simulink model "rlWalkingspotmini_ly"  (R2019a)
settings: Solver=ode113  StartTime=0.0  StopTime=Tf  FixedStep=0.025  RelTol=1e-1  EnableMultiTasking=on
values from neighbouring files (symbols this model uses):
  Tf = 10    [initializeRobotParameters.m]
  Ts = 0.025    [initializeRobotParameters.m]
undefined symbols (not defined in the file or in its folder): height_plane, init_angs_R, init_height, joint_stiffness, plane_x, plane_y, wx0, wy0, X, Y, Z
libraries: sm_lib x66, rlWalkingRobotUtils x20, nesl_utility x14, simulink x5, rllib x1, robotcorelib x1
(part 1 of 3)
settings Model: Creator=The MathWorks, Inc.  LastModifiedBy=liyan
settings SolverCC: ZeroCrossAlgorithm=Adaptive
settings DataIOCC: SaveOutput=off  SignalLogging=off  DSMLogging=off  SaveTime=off  ReturnWorkspaceOutputs=off  OutputTimes=0:0.01:10
settings OptimizationCC: LifeSpan=inf
settings DebuggingCC: AlgebraicLoopMsg=none  MaxConsecutiveZCsMsg=warning  IgnoredZcDiagnostic=none  AllowSymbolicDim=off  SFUnexpectedBacktrackingDiag=warning  SFNoUnconditionalDefaultTransitionDiag=warning  SFExecutionAtInitializationDiag=none  UnitsInconsistencyMsg=none  ArithmeticOperatorsInVariantConditions=warning
settings SFSimCC: SimUseLocalCustomCode=off
settings RTWCC: RTWUseLocalCustomCode=off
settings CodeAppCC: StateflowObjectComments=on
settings GRTTargetCC: TargetLangStandard=C89/C90 (ANSI)  GeneratePreprocessorConditionals=Disable all
settings ConfigComp: CovMetricSettings=dw  CovHtmlReporting=on  CovSaveCumulativeToWorkspaceVar=on  CovSaveSingleToWorkspaceVar=on  CovExternalEMLEnable=off  CovSFcnEnable=off
settings SimscapeCC: SimscapeNormalizeSystem=off  SimscapeLogOpenViewer=on  SimscapeLogLimitData=off  SimscapeLogDataHistory=10000
settings ConfigurationSet: Description=SimMechanics 2G
settings DiagnosticsConfigSet: SimMechanicsRigidlyBoundBlock=none
settings ExplorerConfigSet: InternalSimMechanicsExplorerSettings="<ExplorerConfiguration><canonicalview>default</canonicalview><AnimationSetting><BasePlaybackSpeed>1.0</BasePlaybackSpeed><PlaybackSpeedFactor>1.0</PlaybackSpeedFactor></AnimationSetting><TilePanel><TileInfo><Tiles Columns=\"1\" Count=\"1\" Rows=\"1\"><Column Weight=\"1\"/><Row Weight=\"1\"/><Tile Height=\"1\" Width=\"1\" X=\"0\" Y=\"0\"/></Tiles></TileInfo><SceneInfo><SceneViewer><BGColor><R>0.60000002384185791</R><G>0.60000002384185791</G><B>0.60000002384185791</B></BGColor><Camera><DoPerspective>off</DoPerspective><Position><X>7.18002534815406079</X><Y>-8.21011991112170847</Y><Z>8.33180938462712462</Z></Position><Center><X>1.10741005252516134</X><Y>-0.176829942633513204</Y><Z>0.646464709811595872</Z></Center><Up><X>-0.335329266167064488</X><Y>0.506481739462631531</Y><Z>0.79437430147428989</Z></Up><ViewLimDist>1</ViewLimDist><YLim>0.739205014828661411</YLim><XLim>1.12849377732657596</XLim></Camera></SceneViewer></SceneInfo></TilePanel><MechEditorPanel><Cameras/><GfxPanelCameraMap/><VideoCreator><PlaybackSpeedRatio>1.0</PlaybackSpeedRatio><FrameRate>30</FrameRate><VideoFormat>Motion JPEG AVI</VideoFormat><FrameSize>auto</FrameSize></VideoCreator></MechEditorPanel></ExplorerConfiguration>"

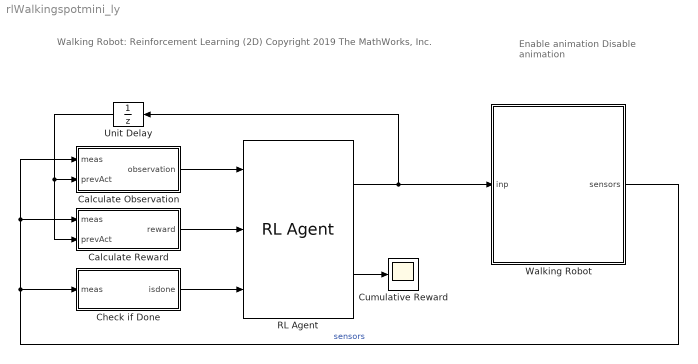
== system rlWalkingspotmini_ly ==
  note: Enable animation
      |
      | Disable animation
  note: Walking Robot: Reinforcement Learning (2D)
      |
      | Copyright 2019 The MathWorks, Inc.
  Calculate Observation : Subsystem
  Calculate Reward : Subsystem
  Check if Done : Subsystem
  Cumulative Reward : Scope
  RL Agent : rllib/RL Agent  Agent=agent  ProvideReward=on  ProvideIsDone=on  ProvideCumRwd=on  TreatAsDirectFeedthrough=on  CollectLoggedSignals=on  CollectModelStates=on
      settings: SourceProductName=Reinforcement Learning Toolbox
  Unit Delay : UnitDelay  SampleTime=-1  HasFrameUpgradeWarning=on
  Walking Robot : Subsystem
  wires:
  Walking Robot/1(sensors) -> Calculate Reward/1(meas), Calculate Observation/1(meas), Check if Done/1(meas)  "sensors"
  Calculate Reward/1(reward) -> RL Agent/2
  Calculate Observation/1(observation) -> RL Agent/1
  Check if Done/1(isdone) -> RL Agent/3
  RL Agent/2 -> Cumulative Reward/1
  Unit Delay/1 -> Calculate Reward/2(prevAct), Calculate Observation/2(prevAct)
  RL Agent/1 -> Walking Robot/1(inp), Unit Delay/1

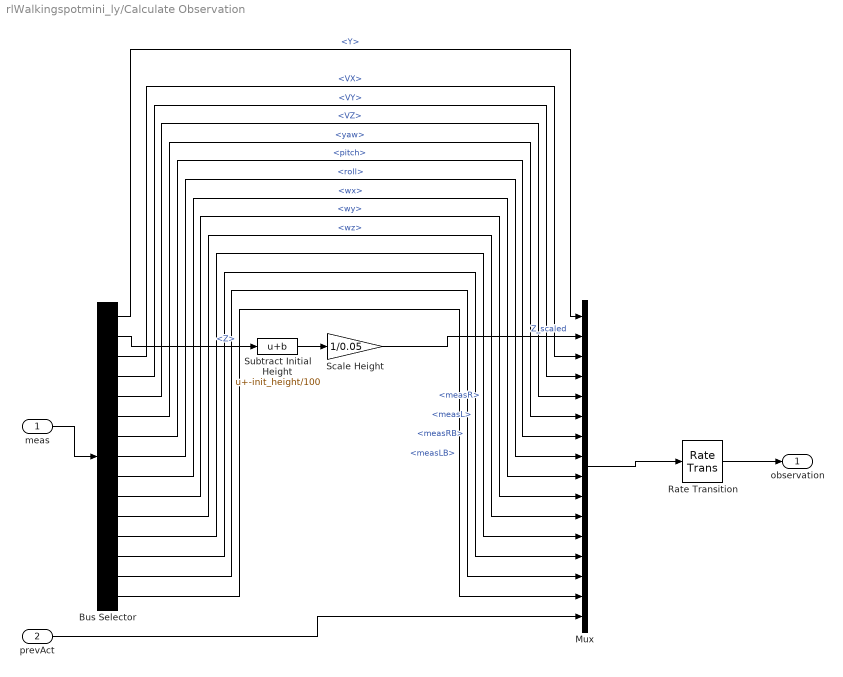
== system rlWalkingspotmini_ly/Calculate Observation ==
  meas : Inport
  prevAct : Inport  Port=2
  Bus Selector : BusSelector  OutputSignals=Y,Z,VX,VY,VZ,yaw,pitch,roll,wx,wy,wz,measR,measL,measRB,measLB
  Mux : Mux  Inputs=16
  Rate Transition : RateTransition
  Scale Height : Gain  Gain=1/0.05
  Subtract Initial Height : Bias  Bias=-init_height/100
  observation : Outport
  wires:
  meas/1 -> Bus Selector/1
  Mux/1 -> Rate Transition/1
  Rate Transition/1 -> observation/1
  Bus Selector/2 -> Subtract Initial Height/1  "<Z>"
  Subtract Initial Height/1 -> Scale Height/1
  Scale Height/1 -> Mux/2  "Z_scaled"
  Bus Selector/1 -> Mux/1  "<Y>"
  Bus Selector/4 -> Mux/4  "<VY>"
  Bus Selector/5 -> Mux/5  "<VZ>"
  Bus Selector/3 -> Mux/3  "<VX>"
  Bus Selector/6 -> Mux/6  "<yaw>"
  Bus Selector/7 -> Mux/7  "<pitch>"
  Bus Selector/8 -> Mux/8  "<roll>"
  Bus Selector/9 -> Mux/9  "<wx>"
  Bus Selector/10 -> Mux/10  "<wy>"
  Bus Selector/11 -> Mux/11  "<wz>"
  prevAct/1 -> Mux/16
  Bus Selector/12 -> Mux/12  "<measR>"
  Bus Selector/13 -> Mux/13  "<measL>"
  Bus Selector/14 -> Mux/14  "<measRB>"
  Bus Selector/15 -> Mux/15  "<measLB>"

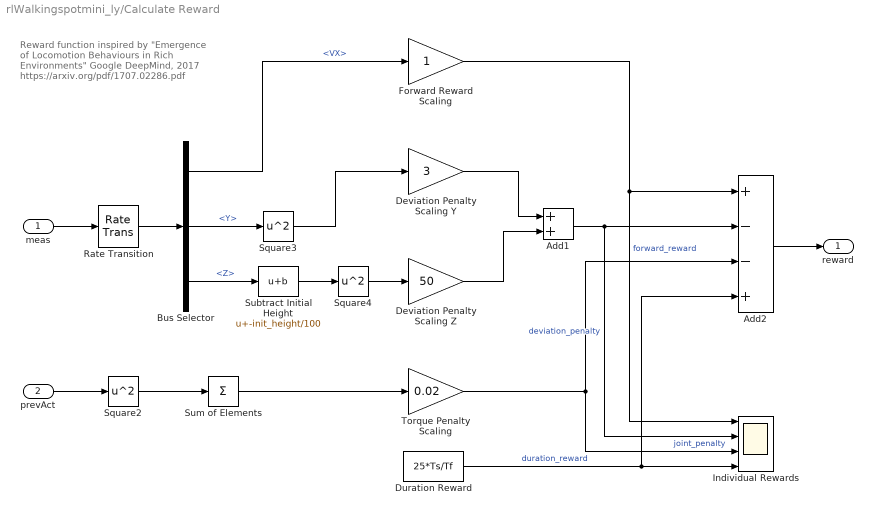
== system rlWalkingspotmini_ly/Calculate Reward ==
  note: Reward function inspired by
      | "Emergence of Locomotion Behaviours in Rich Environments"
      | Google DeepMind, 2017
      | https://arxiv.org/pdf/1707.02286.pdf
  meas : Inport
  prevAct : Inport  Port=2
  Add1 : Sum
  Add2 : Sum  Inputs=+--+
  Bus Selector : BusSelector  OutputSignals=VX,Y,Z
  Deviation Penalty Scaling Y : Gain  Gain=3
  Deviation Penalty Scaling Z : Gain  Gain=50
  Duration Reward : Constant  Value=25*Ts/Tf
  Forward Reward Scaling : Gain
  Individual Rewards : Scope  NumInputPorts=4
  Rate Transition : RateTransition  OutPortSampleTime=Ts
  Square2 : Math  Operator=square  SaturateOnIntegerOverflow=on
  Square3 : Math  Operator=square  SaturateOnIntegerOverflow=on
  Square4 : Math  Operator=square  SaturateOnIntegerOverflow=on
  Subtract Initial Height : Bias  Bias=-init_height/100
  Sum of Elements : Sum  Inputs=+
  Torque Penalty Scaling : Gain  Gain=0.02
  reward : Outport
  wires:
  meas/1 -> Rate Transition/1
  Rate Transition/1 -> Bus Selector/1
  Add2/1 -> reward/1
  Add1/1 -> Add2/2, Individual Rewards/2  "deviation_penalty"
  Forward Reward Scaling/1 -> Add2/1, Individual Rewards/1  "forward_reward"
  Sum of Elements/1 -> Torque Penalty Scaling/1
  Bus Selector/1 -> Forward Reward Scaling/1  "<VX>"
  Bus Selector/2 -> Square3/1  "<Y>"
  Square3/1 -> Deviation Penalty Scaling Y/1
  Duration Reward/1 -> Individual Rewards/4, Add2/4  "duration_reward"
  prevAct/1 -> Square2/1
  Square2/1 -> Sum of Elements/1
  Torque Penalty Scaling/1 -> Add2/3, Individual Rewards/3  "joint_penalty"
  Square4/1 -> Deviation Penalty Scaling Z/1
  Bus Selector/3 -> Subtract Initial Height/1  "<Z>"
  Subtract Initial Height/1 -> Square4/1
  Deviation Penalty Scaling Z/1 -> Add1/2
  Deviation Penalty Scaling Y/1 -> Add1/1

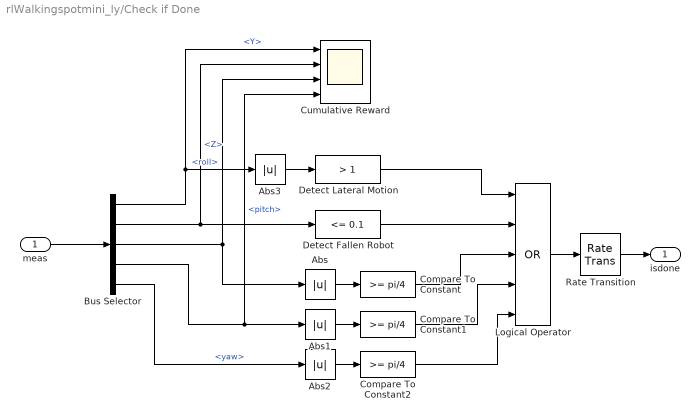
== system rlWalkingspotmini_ly/Check if Done ==
  meas : Inport
  Abs{,1..3} (4 alike) : Abs
  Bus Selector : BusSelector  OutputSignals=Y,Z,roll,pitch,yaw
  Compare To Constant : simulink/Logic and Bit Operations/Compare To Constant  relop=>=  const=pi/4  OutDataTypeStr=boolean
  Compare To Constant1 : simulink/Logic and Bit Operations/Compare To Constant  relop=>=  const=pi/4  OutDataTypeStr=boolean
  Compare To Constant2 : simulink/Logic and Bit Operations/Compare To Constant  relop=>=  const=pi/4  OutDataTypeStr=boolean
  Cumulative Reward : Scope  NumInputPorts=4
  Detect Fallen Robot : simulink/Logic and Bit Operations/Compare To Constant  relop=<=  const=0.1  OutDataTypeStr=boolean
  Detect Lateral Motion : simulink/Logic and Bit Operations/Compare To Constant  relop=>  const=1  OutDataTypeStr=boolean
  Logical Operator : Logic  Operator=OR  Inputs=5  AllPortsSameDT=off  OutDataTypeStr=boolean
  Rate Transition : RateTransition
  isdone : Outport
  wires:
  Logical Operator/1 -> Rate Transition/1
  Bus Selector/2 -> Cumulative Reward/2, Detect Fallen Robot/1  "<Z>"
  meas/1 -> Bus Selector/1
  Detect Fallen Robot/1 -> Logical Operator/2
  Bus Selector/3 -> Abs/1, Cumulative Reward/3  "<roll>"
  Bus Selector/4 -> Cumulative Reward/4, Abs1/1  "<pitch>"
  Compare To Constant/1 -> Logical Operator/3
  Abs/1 -> Compare To Constant/1
  Abs1/1 -> Compare To Constant1/1
  Compare To Constant1/1 -> Logical Operator/4
  Rate Transition/1 -> isdone/1
  Abs2/1 -> Compare To Constant2/1
  Bus Selector/5 -> Abs2/1  "<yaw>"
  Compare To Constant2/1 -> Logical Operator/5
  Abs3/1 -> Detect Lateral Motion/1
  Bus Selector/1 -> Cumulative Reward/1, Abs3/1  "<Y>"
  Detect Lateral Motion/1 -> Logical Operator/1

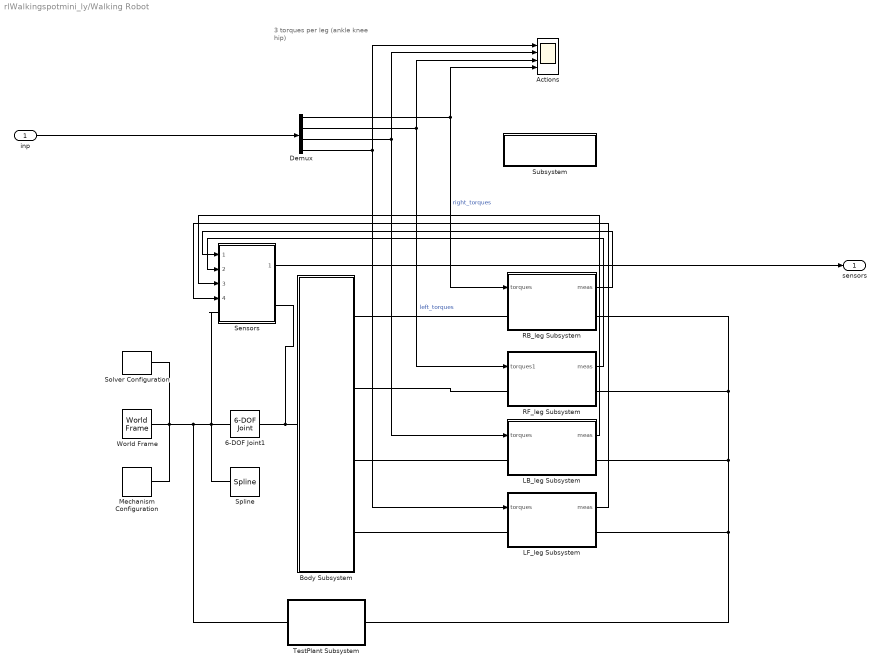
== system rlWalkingspotmini_ly/Walking Robot ==
  note: 3 torques per leg
      | (ankle knee hip)
  inp : Inport
  6-DOF Joint1 : sm_lib/Joints/6-DOF Joint  SenseConstraintForce=off  SenseConstraintForceX=off  SenseConstraintForceY=off  SenseConstraintForceZ=off  SenseConstraintTorque=off  SenseConstraintTorqueX=off  SenseConstraintTorqueY=off  SenseConstraintTorqueZ=off  SenseTotalForce=off  SenseTotalForceX=off  SenseTotalForceY=off  SenseTotalForceZ=off  SenseTotalTorque=off  SenseTotalTorqueX=off  SenseTotalTorqueY=off  SenseTotalTorqueZ=off  CompositeWrenchDir=FollowerOnBase  CompositeWrenchFrame=BaseFrame  PxEquilibriumPosition=0  PxEquilibriumPositionUnits=m  PxSpringStiffness=0  PxSpringStiffnessUnits=N/m  PxDampingCoefficient=world_damping  PxDampingCoefficientUnits=N/(m/s)  PxTorqueActuationMode=NoTorque  PxMotionActuationMode=ComputedMotion  PxSensePosition=off  PxSenseVelocity=off  PxSenseAcceleration=off  PxSenseTorqueForce=off  PxSenseLowerLimitTorqueForce=off  PxSenseUpperLimitTorqueForce=off  PxLowerLimitSpecify=off  PxLowerLimitBound=-1  PxLowerLimitBoundUnits=m  PxLowerLimitStiffness=1e6  PxLowerLimitStiffnessUnits=N/m  PxLowerLimitDamping=1e3  PxLowerLimitDampingUnits=N/(m/s)  PxLowerLimitTransitionRegionWidth=1e-4  PxLowerLimitTransitionRegionWidthUnits=m  PxUpperLimitSpecify=off  PxUpperLimitBound=1  PxUpperLimitBoundUnits=m  PxUpperLimitStiffness=1e6  PxUpperLimitStiffnessUnits=N/m  PxUpperLimitDamping=1e3  PxUpperLimitDampingUnits=N/(m/s)  PxUpperLimitTransitionRegionWidth=1e-4  PxUpperLimitTransitionRegionWidthUnits=m  PxPositionTargetSpecify=on  PxPositionTargetPriority=High  PxPositionTargetValue=0  PxPositionTargetValueUnits=m  PxVelocityTargetSpecify=on  PxVelocityTargetPriority=High  PxVelocityTargetValue=vx0  PxVelocityTargetValueUnits=m/s  PyEquilibriumPosition=0  PyEquilibriumPositionUnits=m  PySpringStiffness=0  PySpringStiffnessUnits=N/m  PyDampingCoefficient=world_damping  PyDampingCoefficientUnits=N/(m/s)  PyTorqueActuationMode=NoTorque  PyMotionActuationMode=ComputedMotion  PySensePosition=off  PySenseVelocity=off  PySenseAcceleration=off  PySenseTorqueForce=off  PySenseLowerLimitTorqueForce=off  PySenseUpperLimitTorqueForce=off  PyLowerLimitSpecify=off  PyLowerLimitBound=-1  PyLowerLimitBoundUnits=m  PyLowerLimitStiffness=1e6  PyLowerLimitStiffnessUnits=N/m  PyLowerLimitDamping=1e3  PyLowerLimitDampingUnits=N/(m/s)  PyLowerLimitTransitionRegionWidth=1e-4  PyLowerLimitTransitionRegionWidthUnits=m  PyUpperLimitSpecify=off  PyUpperLimitBound=1  PyUpperLimitBoundUnits=m  PyUpperLimitStiffness=1e6  PyUpperLimitStiffnessUnits=N/m  PyUpperLimitDamping=1e3  PyUpperLimitDampingUnits=N/(m/s)  PyUpperLimitTransitionRegionWidth=1e-4  PyUpperLimitTransitionRegionWidthUnits=m  PyPositionTargetSpecify=on  PyPositionTargetPriority=High  PyPositionTargetValue=0  PyPositionTargetValueUnits=m  PyVelocityTargetSpecify=on  PyVelocityTargetPriority=High  PyVelocityTargetValue=0  PyVelocityTargetValueUnits=m/s  PzEquilibriumPosition=0  PzEquilibriumPositionUnits=m  PzSpringStiffness=0  PzSpringStiffnessUnits=N/m  PzDampingCoefficient=world_damping  PzDampingCoefficientUnits=N/(m/s)  PzTorqueActuationMode=NoTorque  PzMotionActuationMode=ComputedMotion  PzSensePosition=off  PzSenseVelocity=off  PzSenseAcceleration=off  PzSenseTorqueForce=off  PzSenseLowerLimitTorqueForce=off  PzSenseUpperLimitTorqueForce=off  PzLowerLimitSpecify=off  PzLowerLimitBound=-1  PzLowerLimitBoundUnits=m  PzLowerLimitStiffness=1e6  PzLowerLimitStiffnessUnits=N/m  PzLowerLimitDamping=1e3  PzLowerLimitDampingUnits=N/(m/s)  PzLowerLimitTransitionRegionWidth=1e-4  PzLowerLimitTransitionRegionWidthUnits=m  PzUpperLimitSpecify=off  PzUpperLimitBound=1  PzUpperLimitBoundUnits=m  PzUpperLimitStiffness=1e6  PzUpperLimitStiffnessUnits=N/m  PzUpperLimitDamping=1e3  PzUpperLimitDampingUnits=N/(m/s)  PzUpperLimitTransitionRegionWidth=1e-4  PzUpperLimitTransitionRegionWidthUnits=m  PzPositionTargetSpecify=on  PzPositionTargetPriority=High  PzPositionTargetValue=init_height  PzPositionTargetValueUnits=cm  PzVelocityTargetSpecify=off  PzVelocityTargetPriority=High  PzVelocityTargetValue=0  PzVelocityTargetValueUnits=m/s  SphDefPosRotationMethod=None  SphDefPosRotationAngleUnits=deg  SphDefPosRotationStandardAxis=+Z  SphDefPosRotationAngle=0.0  SphDefPosRotationArbitraryAxis=[0 0 1]  SphDefPosFollAlignAxisA=+X  SphDefPosBaseAlignAxisA=+Y  SphDefPosFollAlignAxisB=+Y  SphDefPosBaseAlignAxisB=+Z  SphDefPosRotationSequenceAxes=FollowerAxes  SphDefPosRotationSequence=XYX  SphDefPosRotationSequenceAngles=[0 0 0]  SphDefPosRotationSequenceAnglesUnits=deg  SphDefPosRotationMatrix=[1 0 0; 0 1 0; 0 0 1]  SphEqPosRotationMethod=None  SphEqPosRotationAngleUnits=deg  SphEqPosRotationStandardAxis=+Z  SphEqPosRotationAngle=0.0  SphEqPosRotationArbitraryAxis=[0 0 1]  SphEqPosFollAlignAxisA=+X  SphEqPosBaseAlignAxisA=+Y  SphEqPosFollAlignAxisB=+Y  SphEqPosBaseAlignAxisB=+Z  SphEqPosRotationSequenceAxes=FollowerAxes  SphEqPosRotationSequence=XYX  SphEqPosRotationSequenceAngles=[0 0 0]  SphEqPosRotationSequenceAnglesUnits=deg  SphEqPosRotationMatrix=[1 0 0; 0 1 0; 0 0 1]  SphSpringStiffness=0  SphSpringStiffnessUnits=N*m/deg  SphDampingCoefficient=world_rot_damping  SphDampingCoefficientUnits=N*m/(rad/s)  SphActuateTorqueX=off  SphActuateTorqueY=off  SphActuateTorqueZ=off  SphActuateTorque=off  SphTorqueActuationMode=NoTorque  SphMotionActuationMode=ComputedMotion  SphActuationFrame=BaseFrame  SphSensePosition=off  SphSenseVelocityX=off  SphSenseVelocityY=off  SphSenseVelocityZ=off  SphSenseVelocity=off  SphSenseAccelerationX=off  SphSenseAccelerationY=off  SphSenseAccelerationZ=off  SphSenseAcceleration=off  SphSenseTorqueX=off  SphSenseTorqueY=off  SphSenseTorqueZ=off  SphSenseTorqueForce=off  SphSenseLowerLimitTorqueMag=off  SphSenseUpperLimitTorqueMag=off  SphSensingFrame=BaseFrame  SphLowerLimitSpecify=off  SphLowerLimitBound=15  SphLowerLimitBoundUnits=deg  SphLowerLimitStiffness=1e4  SphLowerLimitStiffnessUnits=N*m/deg  SphLowerLimitDamping=10  SphLowerLimitDampingUnits=N*m/(deg/s)  SphLowerLimitTransitionRegionWidth=0.1  SphLowerLimitTransitionRegionWidthUnits=deg  SphUpperLimitSpecify=off  SphUpperLimitBound=45  SphUpperLimitBoundUnits=deg  SphUpperLimitStiffness=1e4  SphUpperLimitStiffnessUnits=N*m/deg  SphUpperLimitDamping=10  SphUpperLimitDampingUnits=N*m/(deg/s)  SphUpperLimitTransitionRegionWidth=0.1  SphUpperLimitTransitionRegionWidthUnits=deg  SphPositionTargetRotationMethod=RotationSequence  SphPositionTargetRotationAngleUnits=deg  SphPositionTargetRotationStandardAxis=+Z  SphPositionTargetRotationAngle=0.0  SphPositionTargetRotationArbitraryAxis=[0 0 1]  SphPositionTargetFollAlignAxisA=+X  SphPositionTargetBaseAlignAxisA=+Y  SphPositionTargetFollAlignAxisB=+Y  SphPositionTargetBaseAlignAxisB=+Z  SphPositionTargetRotationSequenceAxes=FollowerAxes  SphPositionTargetRotationSequence=XYX  SphPositionTargetRotationSequenceAngles=[wx0 wy0 0]  SphPositionTargetRotationSequenceAnglesUnits=rad  SphPositionTargetRotationMatrix=eye(3)  SphPositionTargetSpecify=on  SphPositionTargetPriority=High  SphVelocityTargetValue=[0 0 0]  SphVelocityTargetValueUnits=deg/s  SphVelocityTargetSpecify=off  SphVelocityTargetPriority=High  SphVelocityTargetInFollowerFrame=on
  Actions : Scope  NumInputPorts=4
  Body Subsystem : Subsystem
  Demux : Demux
  LB_leg Subsystem : Subsystem
  LF_leg Subsystem : Subsystem
  Mechanism Configuration : sm_lib/Utilities/Mechanism Configuration  UniformGravity=Constant  GravityVector=[0 0 -9.80665]  GravityUnits=m/s^2  LinearizationDelta=0.001
  RB_leg Subsystem : Subsystem
  RF_leg Subsystem : Subsystem
  Sensors : Subsystem
  Solver Configuration : nesl_utility/Solver Configuration  PhysicalDomain=network_engine_domain  SubClassName=solver  LeftPortType=input  RightPortType=generic  Tones=[]  Harmonics=[]  SimulateNoise=off  Profile=off  UseLocalSampling=off  EnableSwitchedLinearOptims=on  FrequencyDomain=off  UseCCode=off  RelTol=0.001  AbsTol=1e-06  MinStep=1e-09  ToWorkspace=off  RevertToSquareIcSolve=off  NumHomotopyIterations=100  PhasorMode=off  PhasorModeNumHarmonics=1  DoDC=off  ResidualTolerance=1e-09  UseLocalSolver=off  LocalSolverChoice=NE_BACKWARD_EULER_ADVANCER  LocalSolverSampleTime=0.001  DoFixedCost=off  MaxNonlinIter=3  MaxModeIter=2  LinearAlgebra=Sparse  EquationFormulation=NE_TIME_EF  DelaysMemoryBudget=1024  AutomaticFiltering=on  FilteringTimeConstant=0.001  PartitionStorageMethod=AS_NEEDED  PartitionMemoryBudget=1024  PartitionMethod=FAST
  Spline : sm_lib/Curves and Surfaces/Spline  DataPoints=[0 0 0.025; 5 0 0.025]  DataPointsUnits=m  EndConditionType=Natural  GraphicType=FromGeometry  MarkerShape=Sphere  MarkerSize=10  GraphicVisPropType=SimpleVisualProperties  GraphicDiffuseColor=[0 0 0]  GraphicSpecularColor=[0.5 0.5 0.5 1.0]  GraphicAmbientColor=[0.15 0.15 0.15 1.0]  GraphicEmissiveColor=[0.0 0.0 0.0 1.0]  GraphicShininess=75  GraphicOpacity=1.0
      settings: SourceProductName=Simscape Multibody
  Subsystem : Subsystem
      settings: OpenFcn=open_system('sm_lib')
      mask Display: disp(sprintf('Open Simscape Multibody\nLibrary'));
  TestPlant Subsystem : Subsystem
  World Frame : sm_lib/Frames and Transforms/World Frame
  sensors : Outport
  wires:
  Demux/3 -> LB_leg Subsystem/1(torques), Actions/2
  Demux/1 -> RB_leg Subsystem/1(torques), Actions/4  "right_torques"
  RF_leg Subsystem/1(meas) -> Sensors/2(measRB)
  Demux/4 -> LF_leg Subsystem/1(torques), Actions/1
  LB_leg Subsystem/1(meas) -> Sensors/3(measLF)
  LF_leg Subsystem/1(meas) -> Sensors/4(measLB)
  Demux/2 -> RF_leg Subsystem/1(torques1), Actions/3  "left_torques"
  Sensors/1(sensors) -> sensors/1
  inp/1 -> Demux/1
  RB_leg Subsystem/1(meas) -> Sensors/1(measRF)
  connections:
  TestPlant Subsystem/RConn1 -- RB_leg Subsystem/RConn1 -- RF_leg Subsystem/RConn1 -- LB_leg Subsystem/RConn1 -- LF_leg Subsystem/RConn1
  TestPlant Subsystem/LConn1 -- World Frame/RConn1 -- Mechanism Configuration/RConn1 -- Solver Configuration/RConn1 -- 6-DOF Joint1/LConn1 -- Spline/LConn1 -- Sensors/LConn1
  Body Subsystem/LConn1 -- 6-DOF Joint1/RConn1 -- Sensors/RConn1
  RB_leg Subsystem/LConn1 -- Body Subsystem/RConn1
  Body Subsystem/RConn4 -- LF_leg Subsystem/LConn1
  RF_leg Subsystem/LConn1 -- Body Subsystem/RConn2
  Body Subsystem/RConn3 -- LB_leg Subsystem/LConn1

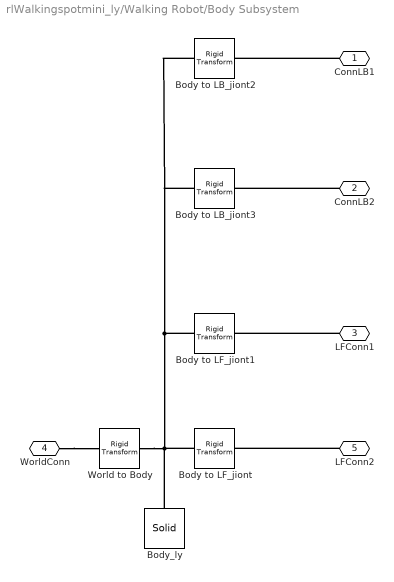
== system rlWalkingspotmini_ly/Walking Robot/Body Subsystem ==
  Body to LB_jiont2 : sm_lib/Frames and Transforms/Rigid Transform  TranslationMethod=Cartesian  TranslationStandardOffset=100  TranslationLengthUnit=mm  TranslationStandardAxis=+Z  TranslationCartesianOffset=[-40 -115 6.5]  TranslationROffset=0  TranslationROffsetUnits=m  TranslationZOffset=0  TranslationZOffsetUnits=m  TranslationThetaOffset=0  TranslationThetaOffsetUnits=deg  RotationMethod=StandardAxis  RotationAngleUnits=deg  RotationStandardAxis=+X  RotationAngle=90  RotationArbitraryAxis=[0 0 1]  FollAlignAxisA=+Z  BaseAlignAxisA=+X  FollAlignAxisB=+Y  BaseAlignAxisB=+Z  RotationSequenceAxes=FollowerAxes  RotationSequence=XYX  RotationSequenceAngles=[0 0 0]  RotationSequenceAnglesUnits=deg  RotationMatrix=[1 0 0; 0 1 0; 0 0 1]
  Body to LB_jiont3 : sm_lib/Frames and Transforms/Rigid Transform  TranslationMethod=Cartesian  TranslationStandardOffset=100  TranslationLengthUnit=mm  TranslationStandardAxis=+Z  TranslationCartesianOffset=[-40 70 6.5]  TranslationROffset=0  TranslationROffsetUnits=m  TranslationZOffset=0  TranslationZOffsetUnits=m  TranslationThetaOffset=0  TranslationThetaOffsetUnits=deg  RotationMethod=StandardAxis  RotationAngleUnits=deg  RotationStandardAxis=+X  RotationAngle=90  RotationArbitraryAxis=[0 0 1]  FollAlignAxisA=+Z  BaseAlignAxisA=+X  FollAlignAxisB=+Y  BaseAlignAxisB=+Z  RotationSequenceAxes=FollowerAxes  RotationSequence=XYX  RotationSequenceAngles=[0 0 0]  RotationSequenceAnglesUnits=deg  RotationMatrix=[1 0 0; 0 1 0; 0 0 1]
  Body to LF_jiont : sm_lib/Frames and Transforms/Rigid Transform  TranslationMethod=Cartesian  TranslationStandardOffset=100  TranslationLengthUnit=mm  TranslationStandardAxis=+Z  TranslationCartesianOffset=[40 70 6.5]  TranslationROffset=0  TranslationROffsetUnits=m  TranslationZOffset=0  TranslationZOffsetUnits=m  TranslationThetaOffset=0  TranslationThetaOffsetUnits=deg  RotationMethod=StandardAxis  RotationAngleUnits=deg  RotationStandardAxis=+X  RotationAngle=90  RotationArbitraryAxis=[0 0 1]  FollAlignAxisA=+Z  BaseAlignAxisA=+X  FollAlignAxisB=+Y  BaseAlignAxisB=+Z  RotationSequenceAxes=FollowerAxes  RotationSequence=XYX  RotationSequenceAngles=[0 0 0]  RotationSequenceAnglesUnits=deg  RotationMatrix=[1 0 0; 0 1 0; 0 0 1]
  Body to LF_jiont1 : sm_lib/Frames and Transforms/Rigid Transform  TranslationMethod=Cartesian  TranslationStandardOffset=100  TranslationLengthUnit=mm  TranslationStandardAxis=+Z  TranslationCartesianOffset=[40 -115 6.5]  TranslationROffset=0  TranslationROffsetUnits=m  TranslationZOffset=0  TranslationZOffsetUnits=m  TranslationThetaOffset=0  TranslationThetaOffsetUnits=deg  RotationMethod=StandardAxis  RotationAngleUnits=deg  RotationStandardAxis=+X  RotationAngle=90  RotationArbitraryAxis=[0 0 1]  FollAlignAxisA=+Z  BaseAlignAxisA=+X  FollAlignAxisB=+Y  BaseAlignAxisB=+Z  RotationSequenceAxes=FollowerAxes  RotationSequence=XYX  RotationSequenceAngles=[0 0 0]  RotationSequenceAnglesUnits=deg  RotationMatrix=[1 0 0; 0 1 0; 0 0 1]
  Body_ly : sm_lib/Body Elements/Solid  InertiaType=Custom  Mass=100  MassUnits=g  CenterOfMass=[0 0 0]  CenterOfMassUnits=mm  MomentsOfInertia=[1 1 1]  MomentsOfInertiaUnits=kg*m^2  ProductsOfInertia=[0 0 0]  ProductsOfInertiaUnits=kg*m^2  BasedOnType=Density  Density=1000  DensityUnits=kg/m^3  DoExposeReferenceFrame=on  SerializedFrames=<Frames/>  GraphicType=FromGeometry  MarkerShape=Sphere  MarkerSize=10  GraphicVisPropType=SimpleVisualProperties  GraphicDiffuseColor=[0.5 0.5 0.5]  GraphicSpecularColor=[0.5 0.5 0.5 1.0]  GraphicAmbientColor=[0.15 0.15 0.15 1.0]  GraphicEmissiveColor=[0.0 0.0 0.0 1.0]  GraphicShininess=75  GraphicOpacity=1.0  GeometryShape=FromFile  RectangleSize=[1 1]  RectangleSizeUnits=m  BrickDimensions=[1 1 1]  BrickDimensionUnits=m  CylinderRadius=1  CylinderRadiusUnits=m  CylinderLength=1  CylinderLengthUnits=m  SphereRadius=1  SphereRadiusUnits=m  EllipsoidRadii=[1 1 1]  EllipsoidRadiiUnits=m  ExtrusionCrossSection=[1 1; -1 1; -1 -1; 1 -1]  ExtrusionCrossSectionUnits=m  ExtrusionLength=1  ExtrusionLengthUnits=m  PolygonNumSides=3  PolygonOuterRadius=1  PolygonOuterRadiusUnits=m  ExtGeomFileType=STL  ExtGeomFileName=D:\MATLAB\robota\sportmicro\sportmicro\body_ly.STL  ExtGeomFileUnits=mm  RevolutionCrossSection=[1 1; 1 -1; 2 -1; 2 1]  RevolutionCrossSectionUnits=m  RevolutionExtent=Full  RevolutionAngle=180  RevolutionAngleUnits=deg
  World to Body : sm_lib/Frames and Transforms/Rigid Transform  TranslationMethod=Cartesian  TranslationStandardOffset=100  TranslationLengthUnit=mm  TranslationStandardAxis=+Z  TranslationCartesianOffset=[0 0 50]  TranslationROffset=0  TranslationROffsetUnits=m  TranslationZOffset=0  TranslationZOffsetUnits=m  TranslationThetaOffset=0  TranslationThetaOffsetUnits=deg  RotationMethod=AlignedAxes  RotationAngleUnits=deg  RotationStandardAxis=+X  RotationAngle=180  RotationArbitraryAxis=[0 0 1]  FollAlignAxisA=+Z  BaseAlignAxisA=-Z  FollAlignAxisB=-X  BaseAlignAxisB=-Y  RotationSequenceAxes=BaseAxes  RotationSequence=XYX  RotationSequenceAngles=[180 0 0]  RotationSequenceAnglesUnits=deg  RotationMatrix=[1 0 0; 0 1 0; 0 0 1]
  ConnLB1 : PMIOPort  Side=Right
  ConnLB2 : PMIOPort  Port=2  Side=Right
  LFConn1 : PMIOPort  Port=3  Side=Right
  WorldConn : PMIOPort  Port=4  Side=Left
  LFConn2 : PMIOPort  Port=5  Side=Right
  connections:
  LFConn2/RConn1 -- Body to LF_jiont/RConn1
  Body_ly/RConn1 -- Body to LB_jiont3/LConn1 -- Body to LB_jiont2/LConn1 -- Body to LF_jiont1/LConn1 -- World to Body/RConn1 -- Body to LF_jiont/LConn1
  LFConn1/RConn1 -- Body to LF_jiont1/RConn1
  WorldConn/RConn1 -- World to Body/LConn1
  ConnLB2/RConn1 -- Body to LB_jiont3/RConn1
  ConnLB1/RConn1 -- Body to LB_jiont2/RConn1

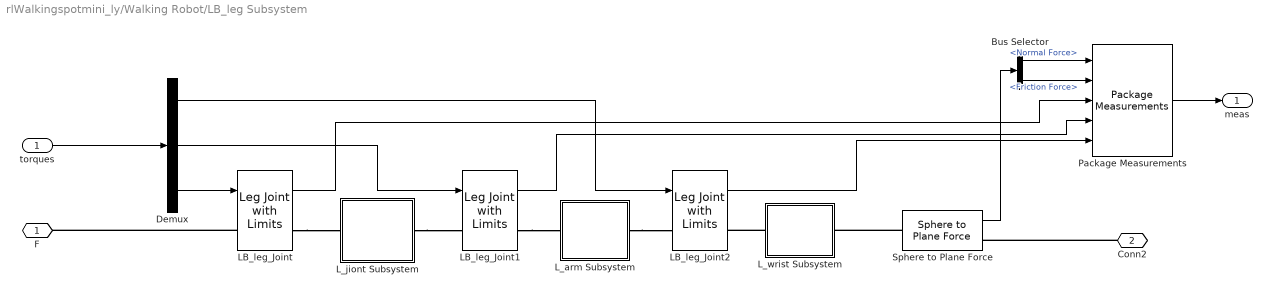
== system rlWalkingspotmini_ly/Walking Robot/LB_leg Subsystem ==
  torques : Inport
  Bus Selector : BusSelector  OutputSignals=Normal Force,Friction Force
  Demux : Demux  Outputs=3
  LB_leg_Joint : rlWalkingRobotUtils/Leg Joint with Limits  VariantControl=actuatorType == 2  k=joint_stiffness  d=joint_damping  initAngle=0%init_angs_R(2)  eqAngle=0  upperLimit=pi  lowerLimit=0  jointLimitStiffness=joint_limit_stiffness  jointLimitDamping=joint_limit_damping
  LB_leg_Joint1 : rlWalkingRobotUtils/Leg Joint with Limits  VariantControl=actuatorType == 2  k=joint_stiffness  d=joint_damping  initAngle=0%init_angs_R(2)  eqAngle=0  upperLimit=pi  lowerLimit=0  jointLimitStiffness=joint_limit_stiffness  jointLimitDamping=joint_limit_damping
  LB_leg_Joint2 : rlWalkingRobotUtils/Leg Joint with Limits  VariantControl=actuatorType == 2  k=joint_stiffness  d=joint_damping  initAngle=0%init_angs_R(2)  eqAngle=0  upperLimit=pi  lowerLimit=0  jointLimitStiffness=joint_limit_stiffness  jointLimitDamping=joint_limit_damping
  L_arm Subsystem : Subsystem
  L_jiont Subsystem : Subsystem
  L_wrist Subsystem : Subsystem
  Package Measurements : rlWalkingRobotUtils/Package  Measurements  SystemSampleTime=-1
  Sphere to Plane Force : rlWalkingRobotUtils/Sphere to Plane Force  sphere_rad=contact_point_radius  plane_lenx=plane_x  plane_leny=plane_y  plane_depth=height_plane/2  force_law=Linear  k_contact=contact_stiffness  b_contact=contact_damping  pen_full_damp_F=1e-4  pen_exponent=1  custom_param_1=1  custom_param_2=1  friction_law=Stick-Slip Continuous  mu_kinetic=mu_k  mu_static=mu_s  v_thr=mu_vth  vis_on=on  vis_opc_en=0  vis_len_plaBz=0.005  vis_clr=[0.9 0.2 0.2]  vis_opc=0.7
  F : PMIOPort  Side=Left
  Conn2 : PMIOPort  Port=2  Side=Right
  meas : Outport
  wires:
  torques/1 -> Demux/1
  Demux/3 -> LB_leg_Joint/1
  Demux/2 -> LB_leg_Joint1/1
  Demux/1 -> LB_leg_Joint2/1
  Bus Selector/1 -> Package Measurements/1  "<Normal Force>"
  Sphere to Plane Force/1 -> Bus Selector/1
  Package Measurements/1 -> meas/1
  Bus Selector/2 -> Package Measurements/2  "<Friction Force>"
  LB_leg_Joint/1 -> Package Measurements/3
  LB_leg_Joint1/1 -> Package Measurements/4
  LB_leg_Joint2/1 -> Package Measurements/5
  connections:
  LB_leg_Joint1/RConn1 -- L_arm Subsystem/LConn1
  L_arm Subsystem/RConn1 -- LB_leg_Joint2/LConn1
  L_jiont Subsystem/RConn1 -- LB_leg_Joint1/LConn1
  L_wrist Subsystem/LConn1 -- LB_leg_Joint2/RConn1
  LB_leg_Joint/LConn1 -- F/RConn1
  LB_leg_Joint/RConn1 -- L_jiont Subsystem/LConn1
  Sphere to Plane Force/LConn1 -- L_wrist Subsystem/RConn1
  Conn2/RConn1 -- Sphere to Plane Force/RConn1

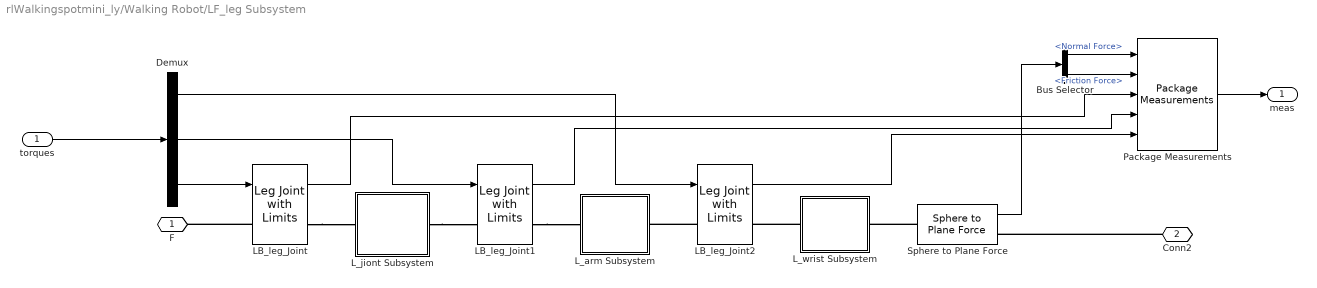
== system rlWalkingspotmini_ly/Walking Robot/LF_leg Subsystem ==
  torques : Inport
  Bus Selector : BusSelector  OutputSignals=Normal Force,Friction Force
  Demux : Demux  Outputs=3
  LB_leg_Joint : rlWalkingRobotUtils/Leg Joint with Limits  VariantControl=actuatorType == 2  k=joint_stiffness  d=joint_damping  initAngle=0%init_angs_R(2)  eqAngle=0  upperLimit=pi  lowerLimit=0  jointLimitStiffness=joint_limit_stiffness  jointLimitDamping=joint_limit_damping
  LB_leg_Joint1 : rlWalkingRobotUtils/Leg Joint with Limits  VariantControl=actuatorType == 2  k=joint_stiffness  d=joint_damping  initAngle=0%init_angs_R(2)  eqAngle=0  upperLimit=pi  lowerLimit=0  jointLimitStiffness=joint_limit_stiffness  jointLimitDamping=joint_limit_damping
  LB_leg_Joint2 : rlWalkingRobotUtils/Leg Joint with Limits  VariantControl=actuatorType == 2  k=joint_stiffness  d=joint_damping  initAngle=0%init_angs_R(2)  eqAngle=0  upperLimit=pi  lowerLimit=0  jointLimitStiffness=joint_limit_stiffness  jointLimitDamping=joint_limit_damping
  L_arm Subsystem : Subsystem
  L_jiont Subsystem : Subsystem
  L_wrist Subsystem : Subsystem
  Package Measurements : rlWalkingRobotUtils/Package  Measurements  SystemSampleTime=-1
  Sphere to Plane Force : rlWalkingRobotUtils/Sphere to Plane Force  sphere_rad=contact_point_radius  plane_lenx=plane_x  plane_leny=plane_y  plane_depth=height_plane/2  force_law=Linear  k_contact=contact_stiffness  b_contact=contact_damping  pen_full_damp_F=1e-4  pen_exponent=1  custom_param_1=1  custom_param_2=1  friction_law=Stick-Slip Continuous  mu_kinetic=mu_k  mu_static=mu_s  v_thr=mu_vth  vis_on=on  vis_opc_en=0  vis_len_plaBz=0.005  vis_clr=[0.9 0.2 0.2]  vis_opc=0.7
  F : PMIOPort  Side=Left
  Conn2 : PMIOPort  Port=2  Side=Right
  meas : Outport
  wires:
  torques/1 -> Demux/1
  Demux/3 -> LB_leg_Joint/1
  Demux/2 -> LB_leg_Joint1/1
  Demux/1 -> LB_leg_Joint2/1
  Bus Selector/1 -> Package Measurements/1  "<Normal Force>"
  Sphere to Plane Force/1 -> Bus Selector/1
  Package Measurements/1 -> meas/1
  Bus Selector/2 -> Package Measurements/2  "<Friction Force>"
  LB_leg_Joint/1 -> Package Measurements/3
  LB_leg_Joint1/1 -> Package Measurements/4
  LB_leg_Joint2/1 -> Package Measurements/5
  connections:
  LB_leg_Joint/LConn1 -- F/RConn1
  L_wrist Subsystem/LConn1 -- LB_leg_Joint2/RConn1
  L_jiont Subsystem/RConn1 -- LB_leg_Joint1/LConn1
  LB_leg_Joint2/LConn1 -- L_arm Subsystem/RConn1
  LB_leg_Joint1/RConn1 -- L_arm Subsystem/LConn1
  LB_leg_Joint/RConn1 -- L_jiont Subsystem/LConn1
  Sphere to Plane Force/LConn1 -- L_wrist Subsystem/RConn1
  Conn2/RConn1 -- Sphere to Plane Force/RConn1

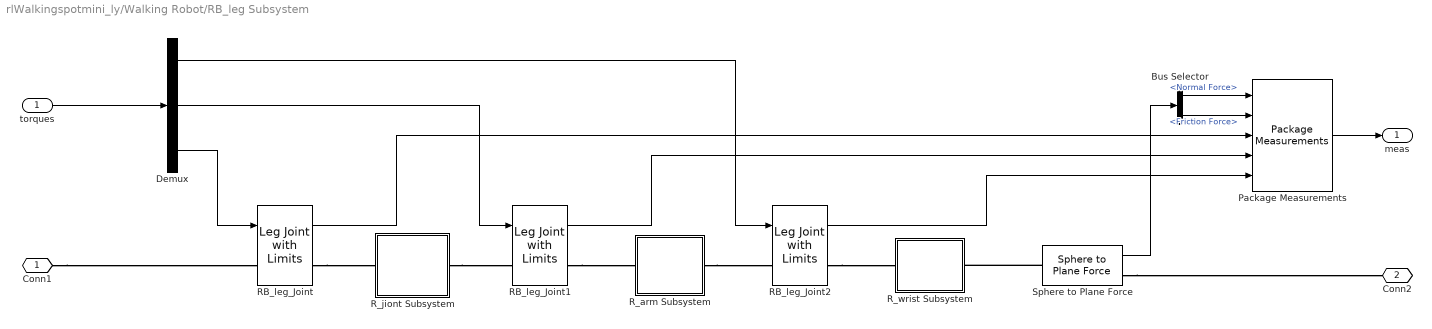
== system rlWalkingspotmini_ly/Walking Robot/RB_leg Subsystem ==
  torques : Inport
  Bus Selector : BusSelector  OutputSignals=Normal Force,Friction Force
  Demux : Demux  Outputs=3
  Package Measurements : rlWalkingRobotUtils/Package  Measurements  SystemSampleTime=-1
  RB_leg_Joint : rlWalkingRobotUtils/Leg Joint with Limits  VariantControl=actuatorType == 2  k=joint_stiffness  d=joint_damping  initAngle=0%init_angs_R(2)  eqAngle=0  upperLimit=pi  lowerLimit=0  jointLimitStiffness=joint_limit_stiffness  jointLimitDamping=joint_limit_damping
  RB_leg_Joint1 : rlWalkingRobotUtils/Leg Joint with Limits  VariantControl=actuatorType == 2  k=joint_stiffness  d=joint_damping  initAngle=0%init_angs_R(2)  eqAngle=0  upperLimit=pi  lowerLimit=0  jointLimitStiffness=joint_limit_stiffness  jointLimitDamping=joint_limit_damping
  RB_leg_Joint2 : rlWalkingRobotUtils/Leg Joint with Limits  VariantControl=actuatorType == 2  k=joint_stiffness  d=joint_damping  initAngle=0%init_angs_R(2)  eqAngle=0  upperLimit=pi  lowerLimit=0  jointLimitStiffness=joint_limit_stiffness  jointLimitDamping=joint_limit_damping
  R_arm Subsystem : Subsystem
  R_jiont Subsystem : Subsystem
  R_wrist Subsystem : Subsystem
  Sphere to Plane Force : rlWalkingRobotUtils/Sphere to Plane Force  sphere_rad=contact_point_radius  plane_lenx=plane_x  plane_leny=plane_y  plane_depth=height_plane/2  force_law=Linear  k_contact=contact_stiffness  b_contact=contact_damping  pen_full_damp_F=1e-4  pen_exponent=1  custom_param_1=1  custom_param_2=1  friction_law=Stick-Slip Continuous  mu_kinetic=mu_k  mu_static=mu_s  v_thr=mu_vth  vis_on=on  vis_opc_en=0  vis_len_plaBz=0.005  vis_clr=[0.9 0.2 0.2]  vis_opc=0.7
  Conn1 : PMIOPort  Side=Left
  Conn2 : PMIOPort  Port=2  Side=Right
  meas : Outport
  wires:
  Demux/3 -> RB_leg_Joint/1
  Demux/2 -> RB_leg_Joint1/1
  Demux/1 -> RB_leg_Joint2/1
  torques/1 -> Demux/1
  Package Measurements/1 -> meas/1
  Sphere to Plane Force/1 -> Bus Selector/1
  Bus Selector/1 -> Package Measurements/1  "<Normal Force>"
  Bus Selector/2 -> Package Measurements/2  "<Friction Force>"
  RB_leg_Joint/1 -> Package Measurements/3
  RB_leg_Joint1/1 -> Package Measurements/4
  RB_leg_Joint2/1 -> Package Measurements/5
  connections:
  RB_leg_Joint1/RConn1 -- R_arm Subsystem/LConn1
  R_arm Subsystem/RConn1 -- RB_leg_Joint2/LConn1
  RB_leg_Joint2/RConn1 -- R_wrist Subsystem/LConn1
  Conn1/RConn1 -- RB_leg_Joint/LConn1
  RB_leg_Joint/RConn1 -- R_jiont Subsystem/LConn1
  R_jiont Subsystem/RConn1 -- RB_leg_Joint1/LConn1
  Sphere to Plane Force/LConn1 -- R_wrist Subsystem/RConn1
  Sphere to Plane Force/RConn1 -- Conn2/RConn1

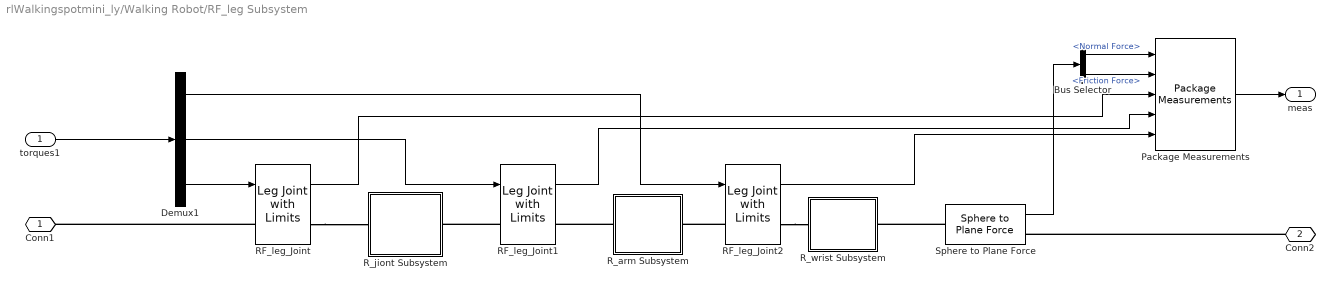
== system rlWalkingspotmini_ly/Walking Robot/RF_leg Subsystem ==
  torques1 : Inport
  Bus Selector : BusSelector  OutputSignals=Normal Force,Friction Force
  Demux1 : Demux  Outputs=3
  Package Measurements : rlWalkingRobotUtils/Package  Measurements  SystemSampleTime=-1
  RF_leg_Joint : rlWalkingRobotUtils/Leg Joint with Limits  VariantControl=actuatorType == 2  k=joint_stiffness  d=joint_damping  initAngle=0%init_angs_R(2)  eqAngle=0  upperLimit=pi  lowerLimit=0  jointLimitStiffness=joint_limit_stiffness  jointLimitDamping=joint_limit_damping
  RF_leg_Joint1 : rlWalkingRobotUtils/Leg Joint with Limits  VariantControl=actuatorType == 2  k=joint_stiffness  d=joint_damping  initAngle=0%init_angs_R(2)  eqAngle=0  upperLimit=pi  lowerLimit=0  jointLimitStiffness=joint_limit_stiffness  jointLimitDamping=joint_limit_damping
  RF_leg_Joint2 : rlWalkingRobotUtils/Leg Joint with Limits  VariantControl=actuatorType == 2  k=joint_stiffness  d=joint_damping  initAngle=0%init_angs_R(2)  eqAngle=0  upperLimit=pi  lowerLimit=0  jointLimitStiffness=joint_limit_stiffness  jointLimitDamping=joint_limit_damping
  R_arm Subsystem : Subsystem
  R_jiont Subsystem : Subsystem
  R_wrist Subsystem : Subsystem
  Sphere to Plane Force : rlWalkingRobotUtils/Sphere to Plane Force  sphere_rad=contact_point_radius  plane_lenx=plane_x  plane_leny=plane_y  plane_depth=height_plane/2  force_law=Linear  k_contact=contact_stiffness  b_contact=contact_damping  pen_full_damp_F=1e-4  pen_exponent=1  custom_param_1=1  custom_param_2=1  friction_law=Stick-Slip Continuous  mu_kinetic=mu_k  mu_static=mu_s  v_thr=mu_vth  vis_on=on  vis_opc_en=0  vis_len_plaBz=0.005  vis_clr=[0.9 0.2 0.2]  vis_opc=0.7
  Conn1 : PMIOPort  Side=Left
  Conn2 : PMIOPort  Port=2  Side=Right
  meas : Outport
  wires:
  torques1/1 -> Demux1/1
  Demux1/3 -> RF_leg_Joint/1
  Demux1/2 -> RF_leg_Joint1/1
  Demux1/1 -> RF_leg_Joint2/1
  Bus Selector/1 -> Package Measurements/1  "<Normal Force>"
  Sphere to Plane Force/1 -> Bus Selector/1
  Package Measurements/1 -> meas/1
  Bus Selector/2 -> Package Measurements/2  "<Friction Force>"
  RF_leg_Joint/1 -> Package Measurements/3
  RF_leg_Joint1/1 -> Package Measurements/4
  RF_leg_Joint2/1 -> Package Measurements/5
  connections:
  RF_leg_Joint/LConn1 -- Conn1/RConn1
  RF_leg_Joint2/RConn1 -- R_wrist Subsystem/LConn1
  RF_leg_Joint1/LConn1 -- R_jiont Subsystem/RConn1
  RF_leg_Joint2/LConn1 -- R_arm Subsystem/RConn1
  R_arm Subsystem/LConn1 -- RF_leg_Joint1/RConn1
  RF_leg_Joint/RConn1 -- R_jiont Subsystem/LConn1
  Sphere to Plane Force/LConn1 -- R_wrist Subsystem/RConn1
  Conn2/RConn1 -- Sphere to Plane Force/RConn1

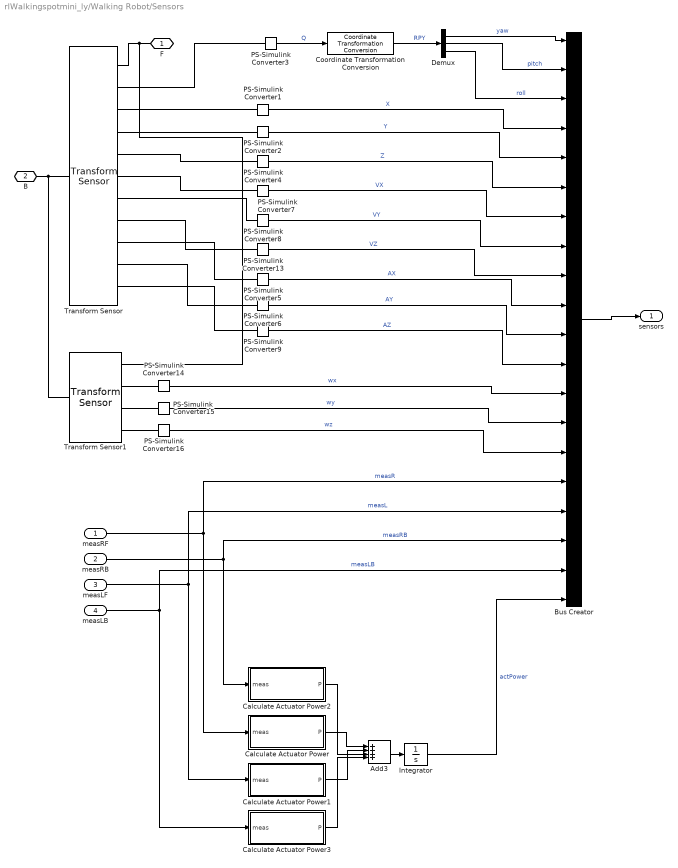
== system rlWalkingspotmini_ly/Walking Robot/Sensors ==
  measRF : Inport
  measRB : Inport  Port=2
  measLF : Inport  Port=3
  measLB : Inport  Port=4
  Add3 : Sum  Inputs=++++
  Bus Creator : BusCreator  Inputs=20
  Calculate Actuator Power : Subsystem
  Calculate Actuator Power1 : Subsystem
  Calculate Actuator Power2 : Subsystem
  Calculate Actuator Power3 : Subsystem
  Coordinate Transformation Conversion : robotcorelib/Coordinate Transformation Conversion  InputRepresentation=Quaternion  InputEulerSequence=ZYX  ShowTrVecInputPort=on  OutputRepresentation=Euler Angles  OutputEulerSequence=ZYX  ShowTrVecOutputPort=on  SimulateUsing=Interpreted execution
      settings: SourceProductBaseCode=RO
  Demux : Demux  Outputs=3
  Integrator : Integrator
  PS-Simulink Converter{1..9,13..16} (13 alike) : nesl_utility/PS-Simulink Converter  PhysicalDomain=network_engine_domain  SubClassName=ps_output  LeftPortType=input  RightPortType=output  PseudoPeriodic=off  Frequencies=[]  Unit=1  AffineConversion=off
  Transform Sensor : sm_lib/Frames and Transforms/Transform Sensor  MeasurementFrame=World  SenseAngle=off  SenseAxis=off  SenseAngle1=off  SenseAngle2=off  SenseAngle3=off  SenseQ=on  SenseR=off  SenseOmegaX=off  SenseOmegaY=off  SenseOmegaZ=off  SenseOmega1=off  SenseOmega2=off  SenseOmega3=off  SenseQDot=off  SenseRDot=off  SenseAlphaX=off  SenseAlphaY=off  SenseAlphaZ=off  SenseAlpha1=off  SenseAlpha2=off  SenseAlpha3=off  SenseQDDot=off  SenseRDDot=off  SenseX=on  SenseY=on  SenseZ=on  SenseRad=off  SenseAzim=off  SenseDist=off  SenseInc=off  SenseXDot=on  SenseYDot=on  SenseZDot=on  SenseRadDot=off  SenseAzimDot=off  SenseDistDot=off  SenseIncDot=off  SenseXDDot=on  SenseYDDot=on  SenseZDDot=on  SenseRadDDot=off  SenseAzimDDot=off  SenseDistDDot=off  SenseIncDDot=off
  Transform Sensor1 : sm_lib/Frames and Transforms/Transform Sensor  MeasurementFrame=NonRotatingFollower  SenseAngle=off  SenseAxis=off  SenseAngle1=off  SenseAngle2=off  SenseAngle3=off  SenseQ=off  SenseR=off  SenseOmegaX=on  SenseOmegaY=on  SenseOmegaZ=on  SenseOmega1=off  SenseOmega2=off  SenseOmega3=off  SenseQDot=off  SenseRDot=off  SenseAlphaX=off  SenseAlphaY=off  SenseAlphaZ=off  SenseAlpha1=off  SenseAlpha2=off  SenseAlpha3=off  SenseQDDot=off  SenseRDDot=off  SenseX=off  SenseY=off  SenseZ=off  SenseRad=off  SenseAzim=off  SenseDist=off  SenseInc=off  SenseXDot=off  SenseYDot=off  SenseZDot=off  SenseRadDot=off  SenseAzimDot=off  SenseDistDot=off  SenseIncDot=off  SenseXDDot=off  SenseYDDot=off  SenseZDDot=off  SenseRadDDot=off  SenseAzimDDot=off  SenseDistDDot=off  SenseIncDDot=off
  F : PMIOPort  Side=Right
  B : PMIOPort  Port=2  Side=Left
  sensors : Outport
  wires:
  PS-Simulink Converter2/1 -> Bus Creator/5  "Y"
  PS-Simulink Converter4/1 -> Bus Creator/6  "Z"
  PS-Simulink Converter5/1 -> Bus Creator/10  "AX"
  Bus Creator/1 -> sensors/1
  PS-Simulink Converter3/1 -> Coordinate Transformation Conversion/1  "Q"
  PS-Simulink Converter1/1 -> Bus Creator/4  "X"
  PS-Simulink Converter6/1 -> Bus Creator/11  "AY"
  PS-Simulink Converter7/1 -> Bus Creator/7  "VX"
  PS-Simulink Converter8/1 -> Bus Creator/8  "VY"
  PS-Simulink Converter9/1 -> Bus Creator/12  "AZ"
  PS-Simulink Converter13/1 -> Bus Creator/9  "VZ"
  Coordinate Transformation Conversion/1 -> Demux/1  "RPY"
  Demux/3 -> Bus Creator/3  "roll"
  Demux/2 -> Bus Creator/2  "pitch"
  Demux/1 -> Bus Creator/1  "yaw"
  PS-Simulink Converter14/1 -> Bus Creator/13  "wx"
  PS-Simulink Converter15/1 -> Bus Creator/14  "wy"
  PS-Simulink Converter16/1 -> Bus Creator/15  "wz"
  measRF/1 -> Calculate Actuator Power/1(meas), Bus Creator/16  "measR"
  measLF/1 -> Bus Creator/17, Calculate Actuator Power1/1(meas)  "measL"
  Calculate Actuator Power/1(P) -> Add3/1
  Calculate Actuator Power1/1(P) -> Add3/2
  Add3/1 -> Integrator/1
  Integrator/1 -> Bus Creator/20  "actPower"
  measRB/1 -> Bus Creator/18, Calculate Actuator Power2/1(meas)  "measRB"
  measLB/1 -> Bus Creator/19, Calculate Actuator Power3/1(meas)  "measLB"
  Calculate Actuator Power2/1(P) -> Add3/3
  Calculate Actuator Power3/1(P) -> Add3/4
  connections:
  PS-Simulink Converter1/LConn1 -- Transform Sensor/RConn3
  PS-Simulink Converter3/LConn1 -- Transform Sensor/RConn2
  Transform Sensor/RConn1 -- Transform Sensor1/RConn1 -- F/RConn1
  Transform Sensor/RConn5 -- PS-Simulink Converter4/LConn1
  Transform Sensor/RConn4 -- PS-Simulink Converter2/LConn1
  Transform Sensor/LConn1 -- Transform Sensor1/LConn1 -- B/RConn1
  PS-Simulink Converter7/LConn1 -- Transform Sensor/RConn6
  PS-Simulink Converter14/LConn1 -- Transform Sensor1/RConn2
  PS-Simulink Converter15/LConn1 -- Transform Sensor1/RConn3
  Transform Sensor1/RConn4 -- PS-Simulink Converter16/LConn1
  Transform Sensor/RConn7 -- PS-Simulink Converter8/LConn1
  PS-Simulink Converter13/LConn1 -- Transform Sensor/RConn8
  PS-Simulink Converter5/LConn1 -- Transform Sensor/RConn9
  Transform Sensor/RConn10 -- PS-Simulink Converter6/LConn1
  PS-Simulink Converter9/LConn1 -- Transform Sensor/RConn11

== system rlWalkingspotmini_ly/Walking Robot/Subsystem ==

== system rlWalkingspotmini_ly/Walking Robot/TestPlant Subsystem ==
  Plane Offset : sm_lib/Frames and Transforms/Rigid Transform  TranslationMethod=StandardAxis  TranslationStandardOffset=height_plane/2  TranslationLengthUnit=m  TranslationStandardAxis=-Z  TranslationCartesianOffset=[0 0 0]  TranslationROffset=0  TranslationROffsetUnits=m  TranslationZOffset=0  TranslationZOffsetUnits=m  TranslationThetaOffset=0  TranslationThetaOffsetUnits=deg  RotationMethod=None  RotationAngleUnits=deg  RotationStandardAxis=+Z  RotationAngle=0.0  RotationArbitraryAxis=[0 0 1]  FollAlignAxisA=+X  BaseAlignAxisA=+Y  FollAlignAxisB=+Y  BaseAlignAxisB=+Z  RotationSequenceAxes=FollowerAxes  RotationSequence=XYX  RotationSequenceAngles=[0 0 0]  RotationSequenceAnglesUnits=deg  RotationMatrix=[1 0 0; 0 1 0; 0 0 1]
  World Plane : sm_lib/Body Elements/Solid  InertiaType=CalculateFromGeometry  Mass=1  MassUnits=kg  CenterOfMass=[0 0 0]  CenterOfMassUnits=m  MomentsOfInertia=[1 1 1]  MomentsOfInertiaUnits=kg*m^2  ProductsOfInertia=[0 0 0]  ProductsOfInertiaUnits=kg*m^2  BasedOnType=Density  Density=density  DensityUnits=kg/(m^3)  DoExposeReferenceFrame=on  SerializedFrames=<Frames/>  GraphicType=FromGeometry  MarkerShape=Sphere  MarkerSize=10  MarkerSizeUnits=m  GraphicVisPropType=SimpleVisualProperties  GraphicDiffuseColor=[1.0 1.0 0.8]  GraphicSpecularColor=[0.5 0.5 0.5 1.0]  GraphicAmbientColor=[0.15 0.15 0.15 1.0]  GraphicEmissiveColor=[0.0 0.0 0.0 1.0]  GraphicShininess=75  GraphicOpacity=0.5  GeometryShape=Brick  RectangleSize=[1 1]  RectangleSizeUnits=m  BrickDimensions="[plane_x plane_y  height_plane]"  BrickDimensionUnits=m  CylinderRadius=1  CylinderRadiusUnits=m  CylinderLength=1  CylinderLengthUnits=m  SphereRadius=1  SphereRadiusUnits=m  EllipsoidRadii=[1 1 1]  EllipsoidRadiiUnits=m  ExtrusionCrossSection=[1 1; -1 1; -1 -1; 1 -1]  ExtrusionCrossSectionUnits=m  ExtrusionLength=1  ExtrusionLengthUnits=m  PolygonNumSides=3  PolygonOuterRadius=1  PolygonOuterRadiusUnits=m  ExtGeomFileType=STL  ExtGeomFileUnits=m  RevolutionCrossSection=[1 1; 1 -1; 2 -1; 2 1]  RevolutionCrossSectionUnits=m  RevolutionExtent=Full  RevolutionAngle=180  RevolutionAngleUnits=deg
  G : PMIOPort  Side=Right
  W : PMIOPort  Port=2  Side=Left
  connections:
  G/RConn1 -- World Plane/RConn1 -- Plane Offset/RConn1
  W/RConn1 -- Plane Offset/LConn1

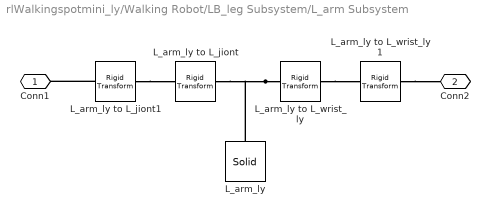
== system rlWalkingspotmini_ly/Walking Robot/LB_leg Subsystem/L_arm Subsystem ==
  L_arm_ly : sm_lib/Body Elements/Solid  InertiaType=Custom  Mass=100  MassUnits=g  CenterOfMass=[10 0 -70]  CenterOfMassUnits=cm  MomentsOfInertia=[1 1 1]  MomentsOfInertiaUnits=kg*m^2  ProductsOfInertia=[0 0 0]  ProductsOfInertiaUnits=kg*m^2  BasedOnType=Mass  Density=1000  DensityUnits=kg/m^3  DoExposeReferenceFrame=on  SerializedFrames=<Frames/>  GraphicType=FromGeometry  MarkerShape=Sphere  MarkerSize=10  GraphicVisPropType=SimpleVisualProperties  GraphicDiffuseColor=[0.5 0.5 0.5]  GraphicSpecularColor=[0.5 0.5 0.5 1.0]  GraphicAmbientColor=[0.15 0.15 0.15 1.0]  GraphicEmissiveColor=[0.0 0.0 0.0 1.0]  GraphicShininess=75  GraphicOpacity=1.0  GeometryShape=FromFile  RectangleSize=[1 1]  RectangleSizeUnits=m  BrickDimensions=[1 1 1]  BrickDimensionUnits=m  CylinderRadius=1  CylinderRadiusUnits=m  CylinderLength=1  CylinderLengthUnits=m  SphereRadius=1  SphereRadiusUnits=m  EllipsoidRadii=[1 1 1]  EllipsoidRadiiUnits=m  ExtrusionCrossSection=[1 1; -1 1; -1 -1; 1 -1]  ExtrusionCrossSectionUnits=m  ExtrusionLength=1  ExtrusionLengthUnits=m  PolygonNumSides=3  PolygonOuterRadius=1  PolygonOuterRadiusUnits=m  ExtGeomFileType=STL  ExtGeomFileName=D:\MATLAB\robota\sportmicro\sportmicro\L_arm_ly.STL  ExtGeomFileUnits=mm  RevolutionCrossSection=[1 1; 1 -1; 2 -1; 2 1]  RevolutionCrossSectionUnits=m  RevolutionExtent=Full  RevolutionAngle=180  RevolutionAngleUnits=deg
  "L_arm_ly to L_wrist_ly " : sm_lib/Frames and Transforms/Rigid Transform  TranslationMethod=None  TranslationStandardOffset=40  TranslationLengthUnit=cm  TranslationStandardAxis=+Y  TranslationCartesianOffset=[-5 0 -8]  TranslationROffset=0  TranslationROffsetUnits=m  TranslationZOffset=0  TranslationZOffsetUnits=m  TranslationThetaOffset=0  TranslationThetaOffsetUnits=deg  RotationMethod=AlignedAxes  RotationAngleUnits=deg  RotationStandardAxis=+X  RotationAngle=90  RotationArbitraryAxis=[0 0 1]  FollAlignAxisA=-Z  BaseAlignAxisA=+Y  FollAlignAxisB=-Y  BaseAlignAxisB=+X  RotationSequenceAxes=FollowerAxes  RotationSequence=XYX  RotationSequenceAngles=[0 0 0]  RotationSequenceAnglesUnits=deg  RotationMatrix=[1 0 0; 0 1 0; 0 0 1]
  L_arm_ly to L_wrist_ly 1 : sm_lib/Frames and Transforms/Rigid Transform  TranslationMethod=None  TranslationStandardOffset=40  TranslationLengthUnit=cm  TranslationStandardAxis=+Y  TranslationCartesianOffset=[-5 0 -8]  TranslationROffset=0  TranslationROffsetUnits=m  TranslationZOffset=0  TranslationZOffsetUnits=m  TranslationThetaOffset=0  TranslationThetaOffsetUnits=deg  RotationMethod=StandardAxis  RotationAngleUnits=deg  RotationStandardAxis=+Z  RotationAngle=90  RotationArbitraryAxis=[0 0 1]  FollAlignAxisA=-Z  BaseAlignAxisA=+Y  FollAlignAxisB=-Y  BaseAlignAxisB=+X  RotationSequenceAxes=FollowerAxes  RotationSequence=XYX  RotationSequenceAngles=[0 0 0]  RotationSequenceAnglesUnits=deg  RotationMatrix=[1 0 0; 0 1 0; 0 0 1]
  "L_arm_ly to L_jiont " : sm_lib/Frames and Transforms/Rigid Transform  TranslationMethod=Cartesian  TranslationStandardOffset=100  TranslationLengthUnit=mm  TranslationStandardAxis=+Z  TranslationCartesianOffset=[15 -28 -105]  TranslationROffset=0  TranslationROffsetUnits=m  TranslationZOffset=0  TranslationZOffsetUnits=m  TranslationThetaOffset=0  TranslationThetaOffsetUnits=deg  RotationMethod=StandardAxis  RotationAngleUnits=deg  RotationStandardAxis=+X  RotationAngle=90  RotationArbitraryAxis=[0 0 1]  FollAlignAxisA=+Z  BaseAlignAxisA=+X  FollAlignAxisB=+Y  BaseAlignAxisB=+Z  RotationSequenceAxes=FollowerAxes  RotationSequence=XYX  RotationSequenceAngles=[0 0 0]  RotationSequenceAnglesUnits=deg  RotationMatrix=[1 0 0; 0 1 0; 0 0 1]
  L_arm_ly to L_jiont1 : sm_lib/Frames and Transforms/Rigid Transform  TranslationMethod=None  TranslationStandardOffset=100  TranslationLengthUnit=cm  TranslationStandardAxis=+Z  TranslationCartesianOffset=[0 0 -50]  TranslationROffset=0  TranslationROffsetUnits=m  TranslationZOffset=0  TranslationZOffsetUnits=m  TranslationThetaOffset=0  TranslationThetaOffsetUnits=deg  RotationMethod=StandardAxis  RotationAngleUnits=deg  RotationStandardAxis=+Y  RotationAngle=180  RotationArbitraryAxis=[0 0 1]  FollAlignAxisA=+Z  BaseAlignAxisA=+X  FollAlignAxisB=+Y  BaseAlignAxisB=+Z  RotationSequenceAxes=FollowerAxes  RotationSequence=XYX  RotationSequenceAngles=[0 0 0]  RotationSequenceAnglesUnits=deg  RotationMatrix=[1 0 0; 0 1 0; 0 0 1]
  Conn1 : PMIOPort  Side=Left
  Conn2 : PMIOPort  Port=2  Side=Right
  connections:
  L_arm_ly to L_wrist_ly 1/RConn1 -- Conn2/RConn1
  L_arm_ly to L_jiont1/LConn1 -- Conn1/RConn1
  "L_arm_ly to L_wrist_ly "/LConn1 -- L_arm_ly/RConn1 -- "L_arm_ly to L_jiont "/LConn1
  "L_arm_ly to L_wrist_ly "/RConn1 -- L_arm_ly to L_wrist_ly 1/LConn1
  L_arm_ly to L_jiont1/RConn1 -- "L_arm_ly to L_jiont "/RConn1
